simulink model "torque_splits"  (R2022b)
settings: Solver=FixedStepAuto  StartTime=0.0  StopTime=0  FixedStep=1  RelTol=1e-3
values from neighbouring files (symbols this model uses):
  dw_MGB = inp.W{3}    [DP_FTP_75.m]
  I_BT_max = (60/t_ch)*I_0    [DP_FTP_75.m]
  P_aux = 0    [DP_FTP_75.m]
  Q_BT_0 = I_0 * 3600    [DP_FTP_75.m]
  Q_BT_in = Q_BT_IC    [DP_FTP_75.m]
  T_CE_cutoff = 5    [DP_FTP_75.m]
  theta_CE = 0.2    [DP_FTP_75.m]
  theta_EM = 0.1    [DP_FTP_75.m]
  Ttot_in = Ttot    [DP_FTP_75.m]
  u1_in = u1    [DP_FTP_75.m]
  u2_in = u2    [DP_FTP_75.m]
  w_CE_idle = 105    [DP_FTP_75.m]
  w_CE_upper = max(w_CE_max)    [DP_FTP_75.m]
  w_EM_upper = max(w_EM_max)    [DP_FTP_75.m]
  w_MGB = wg    [DP_FTP_75.m]
undefined symbols (not defined in the file or in its folder): c_BT_E1, c_BT_E2, c_BT_E3, c_BT_E4, c_BT_L1, c_BT_L2, c_BT_L3, c_BT_L4, eta_EM_map, H_u, I_0, T_CE_max, T_EM_max, V_CE_map, w_CE_max, w_EM_row
libraries: qss_tb_library x1
settings Model: Creator=Jeinil  LastModifiedBy=admin
settings SolverCC: AlgebraicLoopSolver=TrustRegion
settings DataIOCC: ReturnWorkspaceOutputs=off
settings DebuggingCC: UnconnectedInputMsg=warning  UnconnectedOutputMsg=warning  UnconnectedLineMsg=warning  SFMachineParentedDataDiag=warning  ArithmeticOperatorsInVariantConditions=warning
settings ModelReferenceCC: EnableRefExpFcnMdlSchedulingChecks=on
settings SFSimCC: SimUseLocalCustomCode=off  CustomCodeUndefinedFunction=UseInterfaceOnly
settings RTWCC: RTWUseLocalCustomCode=off

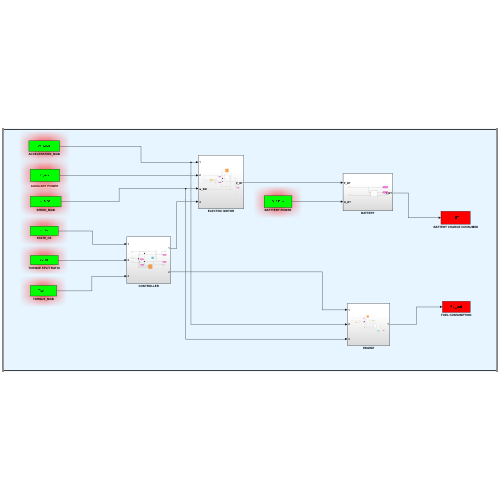
[thumbnail: Simulink's stored preview of the top-level diagram]
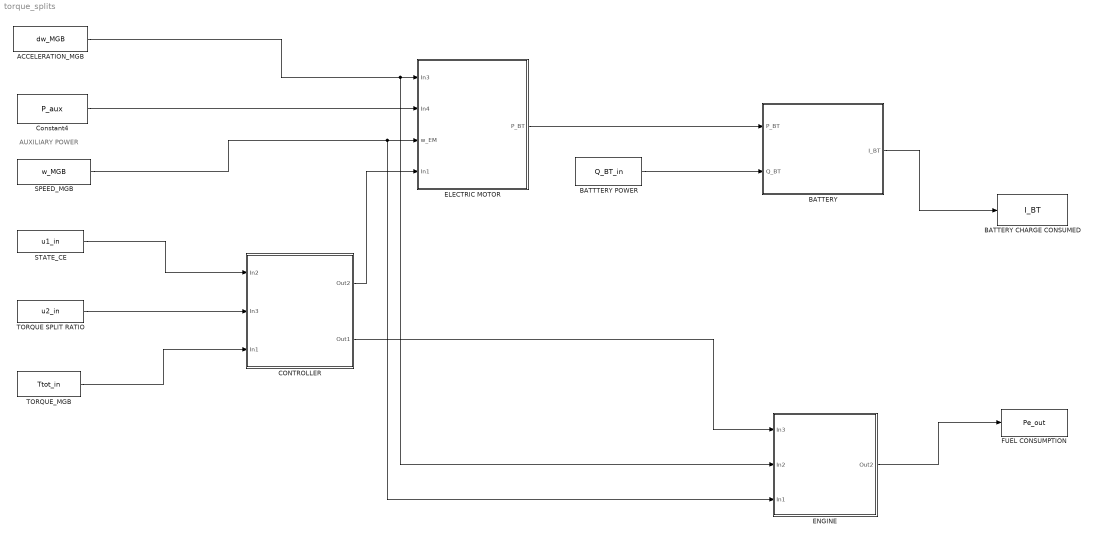
== system torque_splits ==
  note: AUXILIARY POWER
  " BATTERY CHARGE CONSUMED" : ToWorkspace  VariableName=I_BT  SampleTime=-1
  ACCELERATION_MGB : Constant  Value=dw_MGB
  BATTERY : Subsystem
  BATTTERY POWER : Constant  Value=Q_BT_in  SampleTime=-1
  CONTROLLER : Subsystem
  Constant4 : Constant  Value=P_aux
  ELECTRIC MOTOR : Subsystem
  ENGINE : Subsystem
  FUEL CONSUMPTION : ToWorkspace  VariableName=Pe_out  SampleTime=-1
  SPEED_MGB : Constant  Value=w_MGB
  STATE_CE : Constant  Value=u1_in  SampleTime=-1
  TORQUE SPLIT RATIO : Constant  Value=u2_in
  TORQUE_MGB : Constant  Value=Ttot_in  SampleTime=-1
  wires:
  SPEED_MGB/1 -> ENGINE/3(In1), ELECTRIC MOTOR/3(w_EM)
  ACCELERATION_MGB/1 -> ENGINE/2(In2), ELECTRIC MOTOR/1(In3)
  Constant4/1 -> ELECTRIC MOTOR/2(In4)
  ENGINE/1(Out2) -> FUEL CONSUMPTION/1
  CONTROLLER/2(Out1) -> ENGINE/1(In3)
  CONTROLLER/1(Out2) -> ELECTRIC MOTOR/4(In1)
  BATTTERY POWER/1 -> BATTERY/2(Q_BT)
  ELECTRIC MOTOR/1(P_BT) -> BATTERY/1(P_BT)
  BATTERY/1(I_BT) -> " BATTERY CHARGE CONSUMED"/1
  STATE_CE/1 -> CONTROLLER/1(In2)
  TORQUE SPLIT RATIO/1 -> CONTROLLER/2(In3)
  TORQUE_MGB/1 -> CONTROLLER/3(In1)

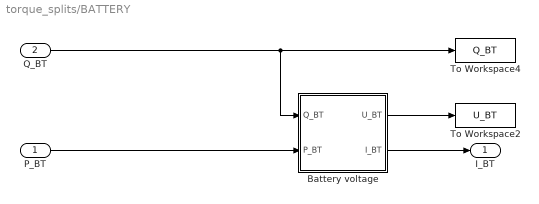
== system torque_splits/BATTERY ==
  P_BT : Inport
  Q_BT : Inport  Port=2
  Battery voltage : Subsystem  AncestorBlock=qss_tb_library/Energy Buffer/Battery/Battery voltage
      settings: LibrarySourceBlock=qss_tb_library/Energy Buffer/Battery/Battery voltage
  To Workspace2 : ToWorkspace  VariableName=U_BT  SampleTime=-1
  To Workspace4 : ToWorkspace  VariableName=Q_BT  SampleTime=-1
  I_BT : Outport
  wires:
  Q_BT/1 -> To Workspace4/1, Battery voltage/1(Q_BT)
  Battery voltage/1(U_BT) -> To Workspace2/1
  Battery voltage/2(I_BT) -> I_BT/1
  P_BT/1 -> Battery voltage/2(P_BT)

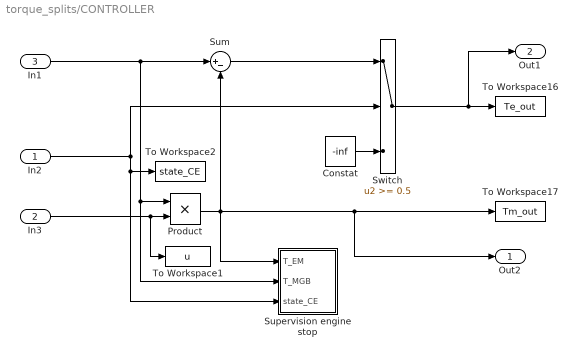
== system torque_splits/CONTROLLER ==
  In2 : Inport
  In3 : Inport  Port=2
  In1 : Inport  Port=3
  Constat : Constant  Value=-inf
  Product : Product  RndMeth=Zero
  Sum : Sum  Inputs=|+-
  Supervision engine stop : Subsystem
  Switch : Switch  Threshold=0.5  SaturateOnIntegerOverflow=off  InputSameDT=off
  To Workspace1 : ToWorkspace  VariableName=u  SampleTime=-1
  To Workspace16 : ToWorkspace  VariableName=Te_out  SampleTime=-1
  To Workspace17 : ToWorkspace  VariableName=Tm_out  SampleTime=-1
  To Workspace2 : ToWorkspace  VariableName=state_CE  SampleTime=-1
  Out2 : Outport
  Out1 : Outport  Port=2
  wires:
  Product/1 -> Out2/1, To Workspace17/1, Supervision engine stop/1(T_EM), Sum/2
  In3/1 -> To Workspace1/1, Product/2
  In1/1 -> Sum/1, Product/1, Supervision engine stop/2(T_MGB)
  Sum/1 -> Switch/1
  Constat/1 -> Switch/3
  In2/1 -> Switch/2, To Workspace2/1, Supervision engine stop/3(state_CE)
  Switch/1 -> Out1/1, To Workspace16/1

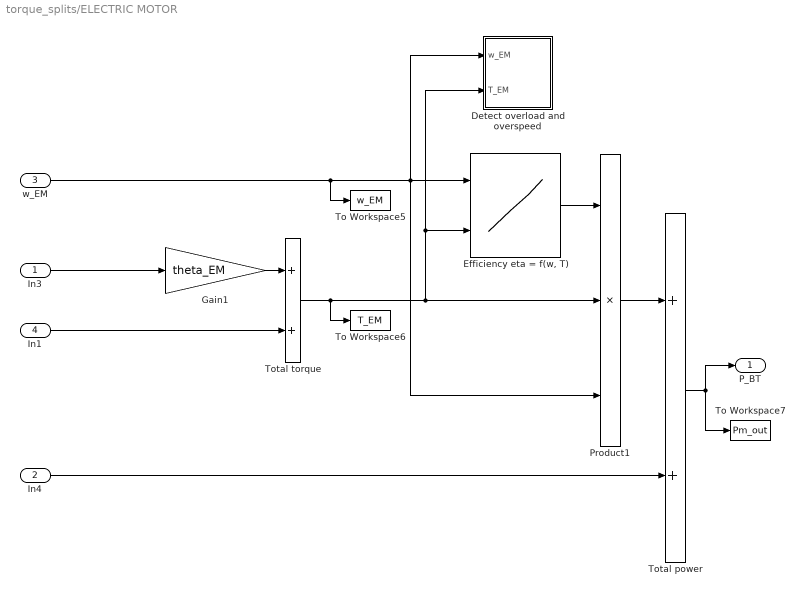
== system torque_splits/ELECTRIC MOTOR ==
  In3 : Inport
  In4 : Inport  Port=2
  w_EM : Inport  Port=3
  In1 : Inport  Port=4
  Detect overload and overspeed : Subsystem  AncestorBlock=|
      | qss_tb_library/Energy Converter/Electric Motor
      | (seminar)/Detect overload
      | and overspeed
      settings: LibrarySourceBlock=|
      | qss_tb_library/Energy Converter/Electric Motor
      | (seminar)/Detect overload
      | and overspeed
  "Efficiency eta = f(w, T)" : Lookup2D  RowIndex=w_EM_row  ColumnIndex=T_EM_col  Table=eta_EM_map  SaturateOnIntegerOverflow=off  InputSameDT=off
  Gain1 : Gain  Gain=theta_EM  SaturateOnIntegerOverflow=on  OutDataTypeStr=Inherit: Same as input  ParamDataTypeStr=Inherit: Same as input
  Product1 : Product  Inputs=3  InputSameDT=on  RndMeth=Zero  SaturateOnIntegerOverflow=on  OutDataTypeStr=Inherit: Same as first input
  To Workspace5 : ToWorkspace  VariableName=w_EM  SampleTime=-1
  To Workspace6 : ToWorkspace  VariableName=T_EM  SampleTime=-1
  To Workspace7 : ToWorkspace  VariableName=Pm_out  SampleTime=-1
  Total power : Sum  InputSameDT=on  SaturateOnIntegerOverflow=on  OutDataTypeStr=Inherit: Same as first input
  Total torque : Sum  InputSameDT=on  SaturateOnIntegerOverflow=on  OutDataTypeStr=Inherit: Same as first input
  P_BT : Outport
  wires:
  Gain1/1 -> Total torque/1
  "Efficiency eta = f(w, T)"/1 -> Product1/1
  In1/1 -> Total torque/2
  w_EM/1 -> To Workspace5/1, Product1/3, "Efficiency eta = f(w, T)"/1, Detect overload and overspeed/1(w_EM)
  Total power/1 -> P_BT/1, To Workspace7/1
  Total torque/1 -> To Workspace6/1, Product1/2, "Efficiency eta = f(w, T)"/2, Detect overload and overspeed/2(T_EM)
  Product1/1 -> Total power/1
  In4/1 -> Total power/2
  In3/1 -> Gain1/1

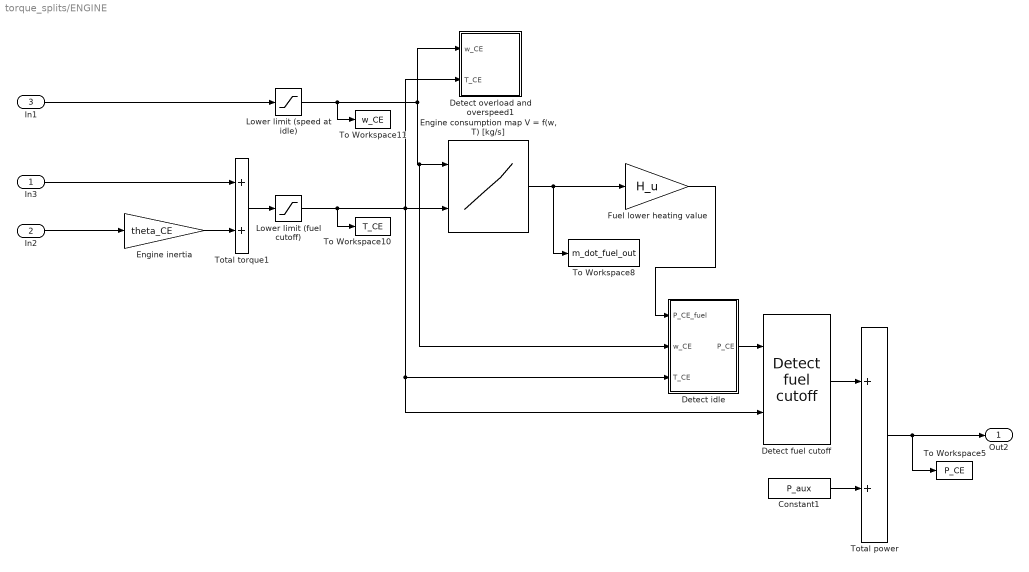
== system torque_splits/ENGINE ==
  In3 : Inport
  In2 : Inport  Port=2
  In1 : Inport  Port=3
  Constant1 : Constant  Value=P_aux
  Detect fuel cutoff : qss_tb_library/Energy Converter/Combustion Engine (consumption map)/Detect fuel cutoff  SystemSampleTime=-1  VariantActivationTime=update diagram  Latency=0  AutoFrameSizeCalculation=off
      link override Constant1: Value=1
      link override Constant3: Value=0
  Detect idle : Subsystem  AncestorBlock=|
      | qss_tb_library/Energy Converter/Combustion Engine
      | (consumption map)/Detect idle
      settings: LibrarySourceBlock=|
      | qss_tb_library/Energy Converter/Combustion Engine
      | (consumption map)/Detect idle
  Detect overload and overspeed1 : Subsystem  AncestorBlock=|
      | qss_tb_library/Energy Converter/Combustion Engine
      | (consumption map)/Detect overload
      | and overspeed
      settings: LibrarySourceBlock=|
      | qss_tb_library/Energy Converter/Combustion Engine
      | (consumption map)/Detect overload
      | and overspeed
  "Engine consumption map V = f(w, T) [kg/s]" : Lookup2D  RowIndex=w_CE_row  ColumnIndex=T_CE_col  Table=V_CE_map  SaturateOnIntegerOverflow=off  InputSameDT=off
  Engine inertia : Gain  Gain=theta_CE  SaturateOnIntegerOverflow=on  OutDataTypeStr=Inherit: Same as input  ParamDataTypeStr=Inherit: Same as input
  Fuel lower heating value : Gain  Gain=H_u  SaturateOnIntegerOverflow=on  OutDataTypeStr=Inherit: Same as input  ParamDataTypeStr=Inherit: Same as input
  Lower limit (fuel cutoff) : Saturate  UpperLimit=inf  LowerLimit=T_CE_cutoff
  Lower limit (speed at idle) : Saturate  UpperLimit=inf  LowerLimit=w_CE_idle
  To Workspace10 : ToWorkspace  VariableName=T_CE  SampleTime=-1
  To Workspace11 : ToWorkspace  VariableName=w_CE  SampleTime=-1
  To Workspace5 : ToWorkspace  VariableName=P_CE  SampleTime=-1
  To Workspace8 : ToWorkspace  VariableName=m_dot_fuel_out  SampleTime=-1
  Total power : Sum  InputSameDT=on  SaturateOnIntegerOverflow=on  OutDataTypeStr=Inherit: Same as first input
  Total torque1 : Sum  InputSameDT=on  SaturateOnIntegerOverflow=on  OutDataTypeStr=Inherit: Same as first input
  Out2 : Outport
  wires:
  Engine inertia/1 -> Total torque1/2
  In2/1 -> Engine inertia/1
  "Engine consumption map V = f(w, T) [kg/s]"/1 -> To Workspace8/1, Fuel lower heating value/1
  Total torque1/1 -> Lower limit (fuel cutoff)/1
  In1/1 -> Lower limit (speed at idle)/1
  In3/1 -> Total torque1/1
  Lower limit (fuel cutoff)/1 -> To Workspace10/1, Detect idle/3(T_CE), Detect fuel cutoff/2, "Engine consumption map V = f(w, T) [kg/s]"/2, Detect overload and overspeed1/2(T_CE)
  Lower limit (speed at idle)/1 -> To Workspace11/1, Detect idle/2(w_CE), "Engine consumption map V = f(w, T) [kg/s]"/1, Detect overload and overspeed1/1(w_CE)
  Detect fuel cutoff/1 -> Total power/1
  Constant1/1 -> Total power/2
  Detect idle/1(P_CE) -> Detect fuel cutoff/1
  Fuel lower heating value/1 -> Detect idle/1(P_CE_fuel)
  Total power/1 -> To Workspace5/1, Out2/1

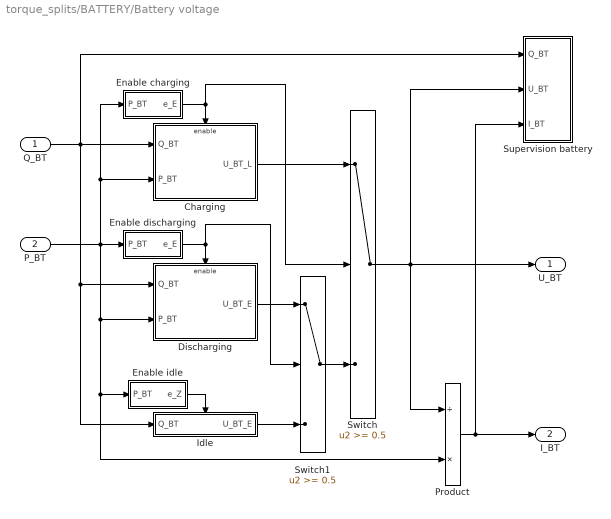
== system torque_splits/BATTERY/Battery voltage ==
  Q_BT : Inport
  P_BT : Inport  Port=2
  Charging : Subsystem
  Discharging : Subsystem
  Enable charging : Subsystem
  Enable discharging : Subsystem
  Enable idle : Subsystem
  Idle : Subsystem
  Product : Product  Inputs=/*  InputSameDT=on  RndMeth=Zero  SaturateOnIntegerOverflow=on  OutDataTypeStr=Inherit: Same as first input
  Supervision battery : Subsystem
  Switch : Switch  Threshold=0.5
  Switch1 : Switch  Threshold=0.5
  U_BT : Outport  InitialOutput=0  VectorParamsAs1DForOutWhenUnconnected=off
  I_BT : Outport  Port=2  InitialOutput=0  VectorParamsAs1DForOutWhenUnconnected=off
  wires:
  Switch/1 -> U_BT/1, Supervision battery/2(U_BT), Product/1
  Enable charging/1(e_E) -> Switch/2, Charging/Enable
  Q_BT/1 -> Idle/1(Q_BT), Discharging/1(Q_BT), Charging/1(Q_BT), Supervision battery/1(Q_BT)
  Product/1 -> I_BT/1, Supervision battery/3(I_BT)
  Enable discharging/1(e_E) -> Switch1/2, Discharging/Enable
  P_BT/1 -> Enable discharging/1(P_BT), Discharging/2(P_BT), Product/2, Enable idle/1(P_BT), Enable charging/1(P_BT), Charging/2(P_BT)
  Discharging/1(U_BT_E) -> Switch1/1
  Idle/1(U_BT_E) -> Switch1/3
  Switch1/1 -> Switch/3
  Charging/1(U_BT_L) -> Switch/1
  Enable idle/1(e_Z) -> Idle/Enable

== system torque_splits/CONTROLLER/Supervision engine stop ==
  T_EM : Inport
  T_MGB : Inport  Port=2
  state_CE : Inport  Port=3
  Interpreted MATLAB Function : MATLABFcn  MATLABFcn=supervision_engine_stop
  Mux : Mux  Inputs=3
  To Workspace : ToWorkspace  VariableName=I1  SampleTime=-1
      settings: Save2DSignal=2-D array (concatenate along first dimension)
  wires:
  T_MGB/1 -> Mux/2
  T_EM/1 -> Mux/1
  state_CE/1 -> Mux/3
  Mux/1 -> Interpreted MATLAB Function/1
  Interpreted MATLAB Function/1 -> To Workspace/1

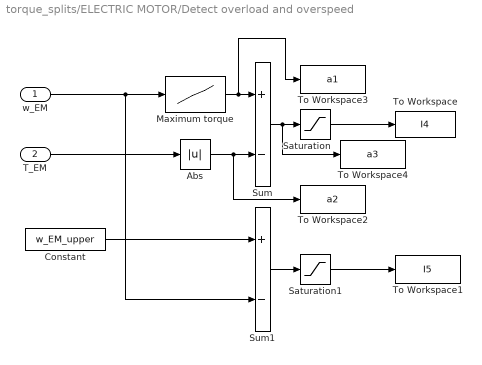
== system torque_splits/ELECTRIC MOTOR/Detect overload and overspeed ==
  w_EM : Inport
  T_EM : Inport  Port=2
  Abs : Abs
  Constant : Constant  Value=w_EM_upper
  Maximum torque : Lookup  InputValues=w_EM_row  Table=T_EM_max
  Saturation : Saturate  UpperLimit=0  LowerLimit=-inf
  Saturation1 : Saturate  UpperLimit=0  LowerLimit=-inf
  Sum : Sum  Inputs=+-  InputSameDT=on  SaturateOnIntegerOverflow=on  OutDataTypeStr=Inherit: Same as first input
  Sum1 : Sum  Inputs=+-  InputSameDT=on  SaturateOnIntegerOverflow=on  OutDataTypeStr=Inherit: Same as first input
  To Workspace : ToWorkspace  VariableName=I4  SampleTime=-1
  To Workspace1 : ToWorkspace  VariableName=I5  SampleTime=-1
      settings: Save2DSignal=2-D array (concatenate along first dimension)
  To Workspace2 : ToWorkspace  VariableName=a2  SampleTime=-1
      settings: Save2DSignal=2-D array (concatenate along first dimension)
  To Workspace3 : ToWorkspace  VariableName=a1  SampleTime=-1
      settings: Save2DSignal=2-D array (concatenate along first dimension)
  To Workspace4 : ToWorkspace  VariableName=a3  SampleTime=-1
      settings: Save2DSignal=2-D array (concatenate along first dimension)
  wires:
  Sum/1 -> To Workspace4/1, Saturation/1
  w_EM/1 -> Maximum torque/1, Sum1/2
  T_EM/1 -> Abs/1
  Maximum torque/1 -> To Workspace3/1, Sum/1
  Abs/1 -> To Workspace2/1, Sum/2
  Saturation/1 -> To Workspace/1
  Constant/1 -> Sum1/1
  Sum1/1 -> Saturation1/1
  Saturation1/1 -> To Workspace1/1

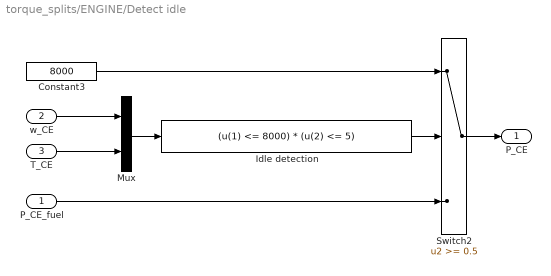
== system torque_splits/ENGINE/Detect idle ==
  P_CE_fuel : Inport
  w_CE : Inport  Port=2
  T_CE : Inport  Port=3
  Constant3 : Constant  Value=8000
  Idle detection : Fcn  Expr=(u(1) <= 8000) * (u(2) <= 5)
  Mux : Mux  Inputs=2
  Switch2 : Switch  Threshold=0.5
  P_CE : Outport  InitialOutput=0
  wires:
  Constant3/1 -> Switch2/1
  Switch2/1 -> P_CE/1
  P_CE_fuel/1 -> Switch2/3
  Idle detection/1 -> Switch2/2
  w_CE/1 -> Mux/1
  T_CE/1 -> Mux/2
  Mux/1 -> Idle detection/1

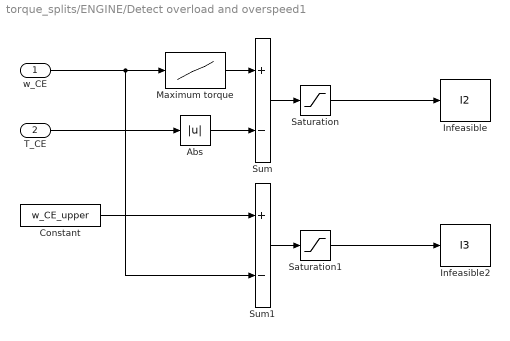
== system torque_splits/ENGINE/Detect overload and overspeed1 ==
  w_CE : Inport
  T_CE : Inport  Port=2
  Abs : Abs
  Constant : Constant  Value=w_CE_upper
  Infeasible : ToWorkspace  VariableName=I2  SampleTime=-1
  Infeasible2 : ToWorkspace  VariableName=I3  SampleTime=-1
  Maximum torque : Lookup  InputValues=w_CE_max  Table=T_CE_max
  Saturation : Saturate  UpperLimit=0  LowerLimit=-inf
  Saturation1 : Saturate  UpperLimit=0  LowerLimit=-inf
  Sum : Sum  Inputs=+-  InputSameDT=on  SaturateOnIntegerOverflow=on  OutDataTypeStr=Inherit: Same as first input
  Sum1 : Sum  Inputs=+-  InputSameDT=on  SaturateOnIntegerOverflow=on  OutDataTypeStr=Inherit: Same as first input
  wires:
  Saturation1/1 -> Infeasible2/1
  Sum1/1 -> Saturation1/1
  Constant/1 -> Sum1/1
  Saturation/1 -> Infeasible/1
  Abs/1 -> Sum/2
  Maximum torque/1 -> Sum/1
  T_CE/1 -> Abs/1
  w_CE/1 -> Sum1/2, Maximum torque/1
  Sum/1 -> Saturation/1

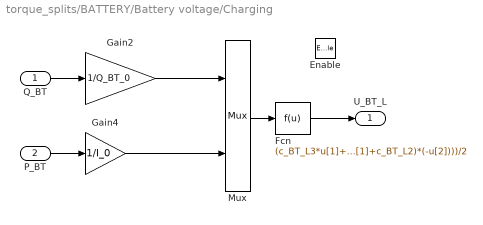
== system torque_splits/BATTERY/Battery voltage/Charging ==
  Q_BT : Inport
  P_BT : Inport  Port=2
  Enable : EnablePort
  Fcn : Fcn  Expr=(c_BT_L3*u[1]+c_BT_L1+sqrt((c_BT_L3*u[1]+c_BT_L1)^2+4*(c_BT_L4*u[1]+c_BT_L2)*(-u[2])))/2
  Gain2 : Gain  Gain=1/Q_BT_0  SaturateOnIntegerOverflow=on  OutDataTypeStr=Inherit: Same as input  ParamDataTypeStr=Inherit: Same as input
  Gain4 : Gain  Gain=1/I_0  SaturateOnIntegerOverflow=on  OutDataTypeStr=Inherit: Same as input  ParamDataTypeStr=Inherit: Same as input
  Mux : Mux  Inputs=2
  U_BT_L : Outport  InitialOutput=0  VectorParamsAs1DForOutWhenUnconnected=off
  wires:
  Fcn/1 -> U_BT_L/1
  Mux/1 -> Fcn/1
  P_BT/1 -> Gain4/1
  Q_BT/1 -> Gain2/1
  Gain2/1 -> Mux/1
  Gain4/1 -> Mux/2

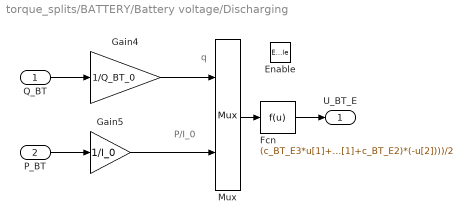
== system torque_splits/BATTERY/Battery voltage/Discharging ==
  note: P/I_0
  note: q
  Q_BT : Inport
  P_BT : Inport  Port=2
  Enable : EnablePort
  Fcn : Fcn  Expr=(c_BT_E3*u[1]+c_BT_E1+sqrt((c_BT_E3*u[1]+c_BT_E1)^2+4*(c_BT_E4*u[1]+c_BT_E2)*(-u[2])))/2
  Gain4 : Gain  Gain=1/Q_BT_0  SaturateOnIntegerOverflow=on  OutDataTypeStr=Inherit: Same as input  ParamDataTypeStr=Inherit: Same as input
  Gain5 : Gain  Gain=1/I_0  SaturateOnIntegerOverflow=on  OutDataTypeStr=Inherit: Same as input  ParamDataTypeStr=Inherit: Same as input
  Mux : Mux  Inputs=2
  U_BT_E : Outport  InitialOutput=0  VectorParamsAs1DForOutWhenUnconnected=off
  wires:
  Mux/1 -> Fcn/1
  Gain5/1 -> Mux/2
  Gain4/1 -> Mux/1
  P_BT/1 -> Gain5/1
  Q_BT/1 -> Gain4/1
  Fcn/1 -> U_BT_E/1

== system torque_splits/BATTERY/Battery voltage/Enable charging ==
  P_BT : Inport
  Gain : Gain  Gain=-1  SaturateOnIntegerOverflow=on  OutDataTypeStr=Inherit: Same as input  ParamDataTypeStr=Inherit: Same as input
  Saturation : Saturate  UpperLimit=0  LowerLimit=-inf
  Sign : Signum
  e_E : Outport  InitialOutput=0  VectorParamsAs1DForOutWhenUnconnected=off
  wires:
  Gain/1 -> Sign/1
  Saturation/1 -> Gain/1
  Sign/1 -> e_E/1
  P_BT/1 -> Saturation/1

== system torque_splits/BATTERY/Battery voltage/Enable discharging ==
  P_BT : Inport
  Saturation : Saturate  UpperLimit=inf  LowerLimit=0
  Sign : Signum
  e_E : Outport  InitialOutput=0  VectorParamsAs1DForOutWhenUnconnected=off
  wires:
  Saturation/1 -> Sign/1
  Sign/1 -> e_E/1
  P_BT/1 -> Saturation/1

== system torque_splits/BATTERY/Battery voltage/Enable idle ==
  P_BT : Inport
  Abs : Abs
  Constant : Constant
  Sign : Signum
  Sum4 : Sum  Inputs=-+  InputSameDT=on  SaturateOnIntegerOverflow=on  OutDataTypeStr=Inherit: Same as first input
  e_Z : Outport  InitialOutput=0  VectorParamsAs1DForOutWhenUnconnected=off
  wires:
  Constant/1 -> Sum4/2
  Sum4/1 -> e_Z/1
  Abs/1 -> Sum4/1
  Sign/1 -> Abs/1
  P_BT/1 -> Sign/1

== system torque_splits/BATTERY/Battery voltage/Idle ==
  Q_BT : Inport
  Enable : EnablePort  StatesWhenEnabling=reset
  Constant : Constant  Value=c_BT_L1
  Gain4 : Gain  Gain=c_BT_L3/Q_BT_0  SaturateOnIntegerOverflow=on  OutDataTypeStr=Inherit: Same as input  ParamDataTypeStr=Inherit: Same as input
  Sum8 : Sum  InputSameDT=on  SaturateOnIntegerOverflow=on  OutDataTypeStr=Inherit: Same as first input
  U_BT_E : Outport  InitialOutput=0  VectorParamsAs1DForOutWhenUnconnected=off
  wires:
  Sum8/1 -> U_BT_E/1
  Constant/1 -> Sum8/2
  Gain4/1 -> Sum8/1
  Q_BT/1 -> Gain4/1

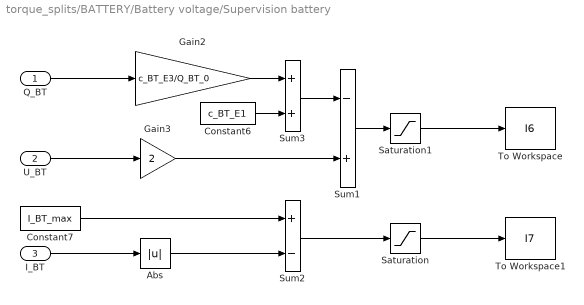
== system torque_splits/BATTERY/Battery voltage/Supervision battery ==
  Q_BT : Inport
  U_BT : Inport  Port=2
  I_BT : Inport  Port=3
  Abs : Abs
  Constant6 : Constant  Value=c_BT_E1
  Constant7 : Constant  Value=I_BT_max
  Gain2 : Gain  Gain=c_BT_E3/Q_BT_0  SaturateOnIntegerOverflow=on  OutDataTypeStr=Inherit: Same as input  ParamDataTypeStr=Inherit: Same as input
  Gain3 : Gain  Gain=2  SaturateOnIntegerOverflow=on  OutDataTypeStr=Inherit: Same as input  ParamDataTypeStr=Inherit: Same as input
  Saturation : Saturate  UpperLimit=0  LowerLimit=-inf
  Saturation1 : Saturate  UpperLimit=0  LowerLimit=-inf
  Sum1 : Sum  Inputs=-+  InputSameDT=on  SaturateOnIntegerOverflow=on  OutDataTypeStr=Inherit: Same as first input
  Sum2 : Sum  Inputs=+-  InputSameDT=on  SaturateOnIntegerOverflow=on  OutDataTypeStr=Inherit: Same as first input
  Sum3 : Sum  InputSameDT=on  SaturateOnIntegerOverflow=on  OutDataTypeStr=Inherit: Same as first input
  To Workspace : ToWorkspace  VariableName=I6  SampleTime=-1
      settings: Save2DSignal=2-D array (concatenate along first dimension)
  To Workspace1 : ToWorkspace  VariableName=I7  SampleTime=-1
      settings: Save2DSignal=2-D array (concatenate along first dimension)
  wires:
  Q_BT/1 -> Gain2/1
  Abs/1 -> Sum2/2
  I_BT/1 -> Abs/1
  Sum2/1 -> Saturation/1
  Constant7/1 -> Sum2/1
  Gain2/1 -> Sum3/1
  Constant6/1 -> Sum3/2
  Sum1/1 -> Saturation1/1
  Saturation1/1 -> To Workspace/1
  Saturation/1 -> To Workspace1/1
  Gain3/1 -> Sum1/2
  U_BT/1 -> Gain3/1
  Sum3/1 -> Sum1/1
